simulink model "Solar_Position"  (R2024b)
settings: Solver=FixedStepAuto  StartTime=0.0  StopTime=1200  FixedStep=0.1  RelTol=1e-3
values from neighbouring files (symbols this model uses):
  DayNum = 0    [Inititialisation.m]
  EGlobal = t(2:25, 2:end)    [Inititialisation.m]
  Latitude = 0    [Inititialisation.m]
  Longitude = 0    [Inititialisation.m]
  T_avg = transpose(t(30,2:end))    [Inititialisation.m]
  TimeDiff = 0    [Inititialisation.m]
libraries: simulink_extras x14
settings Model: Creator=Harrison  LastModifiedBy=Harrison
settings DebuggingCC: AlgebraicLoopMsg=none

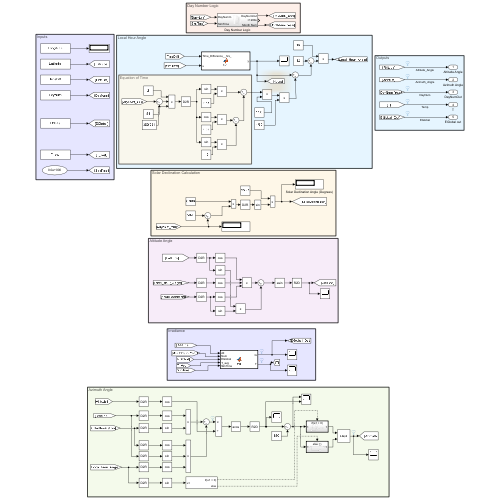
[thumbnail: Simulink's stored preview of the top-level diagram]
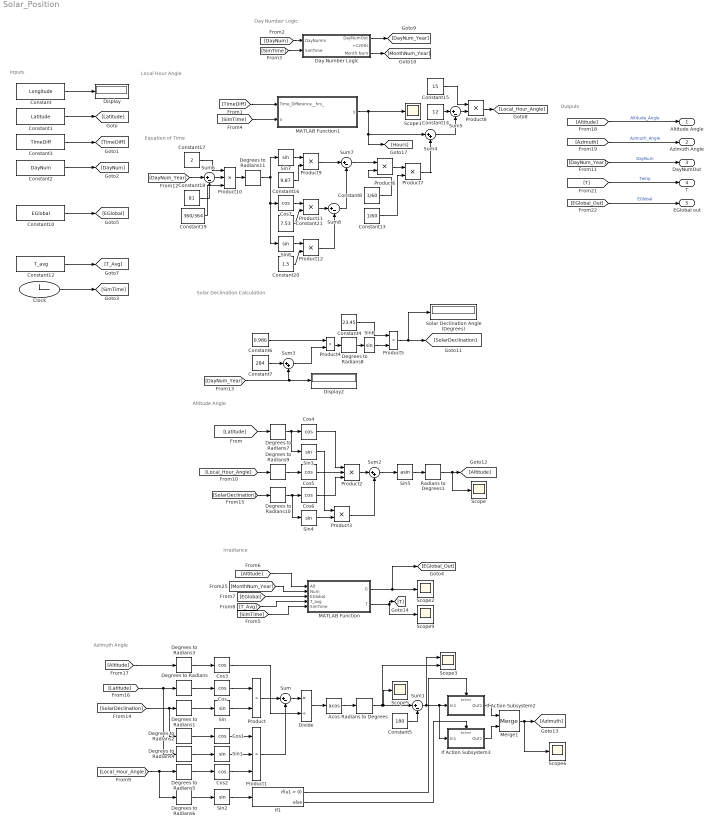
== system Solar_Position ==
  note: Irradiance
  note: Equation of Time
  note: Local Hour Angle
  note: Solar Declination Calculation
  note: Day Number Logic
  note: Altitude Angle
  note: Azimuth Angle
  note: Outputs
  note: Inputs
  Acos : Trigonometry  Operator=acos
  Clock : Clock
      settings: Decimation=100
  Constant : Constant  Value=Longitude
  Constant1 : Constant  Value=Latitude
  Constant10 : Constant  Value=EGlobal
  Constant12 : Constant  Value=T_avg
  Constant13 : Constant  Value=1/60
  Constant14 : Constant  Value=12
  Constant15 : Constant  Value=15
  Constant16 : Constant  Value=9.87
  Constant17 : Constant  Value=2
  Constant18 : Constant  Value=81
  Constant19 : Constant  Value=360/364
  Constant2 : Constant  Value=DayNum
  Constant20 : Constant  Value=1.5
  Constant21 : Constant  Value=7.53
  Constant3 : Constant  Value=TimeDiff
  Constant4 : Constant  Value=23.45
  Constant5 : Constant  Value=180
  Constant6 : Constant  Value=0.986
  Constant7 : Constant  Value=284
  Constant8 : Constant  Value=1/60
  Cos{,1..7} (8 alike) : Trigonometry  Operator=cos
  Day Number Logic : Subsystem
  Degrees to Radians{,1..11} (12 alike) : simulink_extras/Transformations/Degrees to Radians
  Display : Display
  Display2 : Display
  Divide : Product  Inputs=*/
  If Action Subsystem2 : Subsystem  TreatAsAtomicUnit=on
  If Action Subsystem3 : Subsystem  TreatAsAtomicUnit=on
  If1 : If
  MATLAB Function : MATLAB Function  TreatAsAtomicUnit=on
  MATLAB Function1 : MATLAB Function  TreatAsAtomicUnit=on
  Merge1 : Merge
  Product{,3..9,11..12} (10 alike) : Product
  Product1 : Product  Inputs=3
  Product10 : Product  Inputs=3
  Product2 : Product  Inputs=3
  Radians to Degrees : simulink_extras/Transformations/Radians to Degrees
  Radians to Degrees1 : simulink_extras/Transformations/Radians to Degrees
  Scope{,1..2,5..6,9} (6 alike) : Scope
  Scope3 : Scope  NumInputPorts=2
  Sin{,1..4,6..8} (8 alike) : Trigonometry
  Sin5 : Trigonometry  Operator=asin
  Solar Declination Angle (Degrees) : Display
  Sum{,1,5..8} (6 alike) : Sum  Inputs=|+-
  Sum2 : Sum  Inputs=|++
  Sum3 : Sum  Inputs=|++
  Sum4 : Sum  Inputs=|++
  Altitude Angle : Outport
  Azimuth Angle : Outport  Port=2
  DayNumOut : Outport  Port=3
  T : Outport  Port=4
  EGlobal out : Outport  Port=5
  wires:
  Constant/1 -> Display/1
  Radians to Degrees1/1 -> Scope/1, [Altitude]
  Merge1/1 -> Scope6/1, [Azimuth]
  Day Number Logic/1(DayNumOut) -> [DayNum_Year]
  Constant2/1 -> [DayNum]
  MATLAB Function/1(G) -> [EGlobal_Out], Scope2/1
  Constant1/1 -> [Latitude]
  Constant3/1 -> [TimeDiff]
  [DayNum] -> Day Number Logic/1(DayNumIn)
  Clock/1 -> [SimTime]
  [SimTime] -> Day Number Logic/2(SimTime)
  Constant10/1 -> [EGlobal]
  Constant12/1 -> [T_Avg]
  Day Number Logic/3(Month Num) -> [MonthNum_Year]
  [DayNum_Year] -> DayNumOut/1  "DayNum"
  Product8/1 -> [Local_Hour_Angle]
  [Altitude] -> Altitude Angle/1  "Altitude_Angle"
  [Azimuth] -> Azimuth Angle/1  "Azimuth_Angle"
  MATLAB Function/2(T) -> Scope9/1, [T]
  [T] -> T/1  "Temp"
  [EGlobal_Out] -> EGlobal out/1  "EGlobal"
  Degrees to Radians6/1 -> Sin2/1
  Degrees to Radians5/1 -> Cos2/1
  Degrees to Radians4/1 -> Sin1/1
  Degrees to Radians2/1 -> Cos1/1
  Degrees to Radians1/1 -> Sin/1
  Degrees to Radians/1 -> Cos/1
  Constant5/1 -> Sum1/2
  Product/1 -> Sum/1
  Sin/1 -> Product/2
  Cos/1 -> Product/1
  Acos/1 -> Radians to Degrees/1
  Sin1/1 -> Product1/2
  Divide/1 -> Acos/1
  Degrees to Radians3/1 -> Cos3/1
  Sin2/1 -> If1/1
  Cos3/1 -> Divide/2
  Sum/1 -> Divide/1
  If Action Subsystem3/1(Out1) -> Merge1/2
  Cos1/1 -> Product1/1
  Cos2/1 -> Product1/3
  Product1/1 -> Sum/2
  Sum1/1 -> Scope3/1, If Action Subsystem3/1(In1), If Action Subsystem2/1(In1)
  Radians to Degrees/1 -> Sum1/1, Scope5/1, Scope3/2
  If Action Subsystem2/1(Out1) -> Merge1/1
  If1/1 -> If Action Subsystem2/Action
  If1/2 -> If Action Subsystem3/Action
  Degrees to Radians10/1 -> Cos6/1, Sin4/1
  Degrees to Radians9/1 -> Cos5/1
  Degrees to Radians7/1 -> Sin3/1, Cos4/1
  [Local_Hour_Angle] -> Degrees to Radians9/1
  Sum2/1 -> Sin5/1
  Product2/1 -> Sum2/1
  Sin5/1 -> Radians to Degrees1/1
  Product3/1 -> Sum2/2
  Cos6/1 -> Product2/3
  Sin4/1 -> Product3/2
  [Latitude] -> Degrees to Radians7/1
  Sin3/1 -> Product3/1
  Cos5/1 -> Product2/2
  [SolarDeclination] -> Degrees to Radians10/1
  Cos4/1 -> Product2/1
  Sin6/1 -> Product5/2
  Product4/1 -> Degrees to Radians8/1
  Degrees to Radians8/1 -> Sin6/1
  Sum3/1 -> Product4/2
  Constant4/1 -> Product5/1
  Constant6/1 -> Product4/1
  [DayNum_Year] -> Display2/1, Sum3/2
  Constant7/1 -> Sum3/1
  Product5/1 -> Solar Declination Angle (Degrees)/1, [SolarDeclination]
  Sum4/1 -> Sum5/2
  Constant13/1 -> Product7/2
  Product6/1 -> Product7/1
  Sum7/1 -> Product6/1
  Sum5/1 -> Product8/2
  MATLAB Function1/1(y) -> Scope1/1, [Hours], Sum4/1
  Constant14/1 -> Sum5/1
  Product7/1 -> Sum4/2
  Constant8/1 -> Product6/2
  [SimTime] -> MATLAB Function1/2(u)
  Constant15/1 -> Product8/1
  [TimeDiff] -> MATLAB Function1/1(Time_Difference__hrs_)
  [DayNum_Year] -> Sum6/1
  Constant17/1 -> Product10/1
  Product9/1 -> Sum7/1
  Product12/1 -> Sum8/2
  Constant18/1 -> Sum6/2
  Sum6/1 -> Product10/2
  Sin7/1 -> Product9/1
  Product10/1 -> Degrees to Radians11/1
  Sum8/1 -> Sum7/2
  Constant16/1 -> Product9/2
  Cos7/1 -> Product11/1
  Constant21/1 -> Product11/2
  Product11/1 -> Sum8/1
  Degrees to Radians11/1 -> Sin8/1, Cos7/1, Sin7/1
  Constant20/1 -> Product12/2
  Sin8/1 -> Product12/1
  Constant19/1 -> Product10/3
  [SimTime] -> MATLAB Function/5(SimTime)
  [T_Avg] -> MATLAB Function/4(T_avg)
  [EGlobal] -> MATLAB Function/3(EGlobal)
  [MonthNum_Year] -> MATLAB Function/2(Num)
  [Altitude] -> MATLAB Function/1(Alt)
  [SolarDeclination] -> Degrees to Radians2/1, Degrees to Radians1/1
  [Local_Hour_Angle] -> Degrees to Radians6/1, Degrees to Radians5/1
  [Altitude] -> Degrees to Radians3/1
  [Latitude] -> Degrees to Radians4/1, Degrees to Radians/1

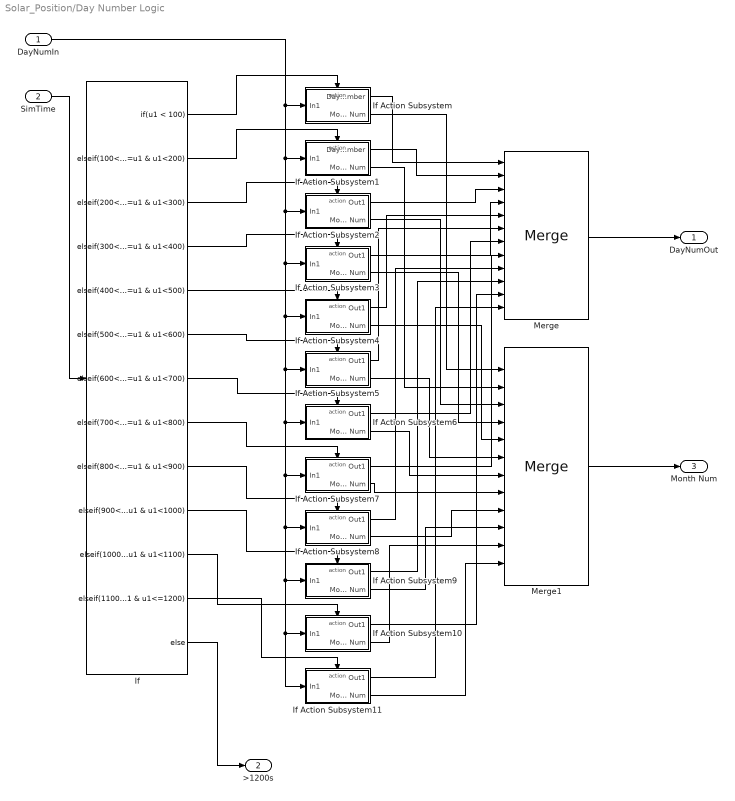
== system Solar_Position/Day Number Logic ==
  DayNumIn : Inport
  SimTime : Inport  Port=2
  If : If  IfExpression=u1 < 100  ElseIfExpressions=100<=u1 & u1<200, 200<=u1 & u1<300, 300<=u1 & u1<400, 400<=u1 & u1<500, 500<=u1 & u1<600, 600<=u1 & u1<700, 700<=u1 & u1<800, 800<=u1 & u1<900, 900<=u1 & u1<1000, 1000<=u1 & u1<1100, 1100<=u1 & u1<=1200
  If Action Subsystem : Subsystem  TreatAsAtomicUnit=on
  If Action Subsystem1 : Subsystem  TreatAsAtomicUnit=on
  If Action Subsystem10 : Subsystem  TreatAsAtomicUnit=on
  If Action Subsystem11 : Subsystem  TreatAsAtomicUnit=on
  If Action Subsystem2 : Subsystem  TreatAsAtomicUnit=on
  If Action Subsystem3 : Subsystem  TreatAsAtomicUnit=on
  If Action Subsystem4 : Subsystem  TreatAsAtomicUnit=on
  If Action Subsystem5 : Subsystem  TreatAsAtomicUnit=on
  If Action Subsystem6 : Subsystem  TreatAsAtomicUnit=on
  If Action Subsystem7 : Subsystem  TreatAsAtomicUnit=on
  If Action Subsystem8 : Subsystem  TreatAsAtomicUnit=on
  If Action Subsystem9 : Subsystem  TreatAsAtomicUnit=on
  Merge : Merge  Inputs=12
  Merge1 : Merge  Inputs=12
  DayNumOut : Outport
  >1200s : Outport  Port=2
  Month Num : Outport  Port=3
  wires:
  If/8 -> If Action Subsystem7/Action
  If/5 -> If Action Subsystem4/Action
  DayNumIn/1 -> If Action Subsystem11/1(In1), If Action Subsystem10/1(In1), If Action Subsystem9/1(In1), If Action Subsystem8/1(In1), If Action Subsystem7/1(In1), If Action Subsystem6/1(In1), If Action Subsystem5/1(In1), If Action Subsystem4/1(In1), If Action Subsystem3/1(In1), If Action Subsystem2/1(In1), If Action Subsystem1/1(In1), If Action Subsystem/1(In1)
  If Action Subsystem/1(Day number) -> Merge/1
  If Action Subsystem10/1(Out1) -> Merge/11
  If Action Subsystem5/1(Out1) -> Merge/6
  If Action Subsystem11/1(Out1) -> Merge/12
  If Action Subsystem8/1(Out1) -> Merge/9
  If/10 -> If Action Subsystem9/Action
  If Action Subsystem6/1(Out1) -> Merge/7
  If/7 -> If Action Subsystem6/Action
  If/11 -> If Action Subsystem10/Action
  If/1 -> If Action Subsystem/Action
  If Action Subsystem7/1(Out1) -> Merge/8
  If/3 -> If Action Subsystem2/Action
  If/12 -> If Action Subsystem11/Action
  If Action Subsystem2/1(Out1) -> Merge/3
  If/6 -> If Action Subsystem5/Action
  If Action Subsystem4/1(Out1) -> Merge/5
  If/2 -> If Action Subsystem1/Action
  If Action Subsystem9/1(Out1) -> Merge/10
  If Action Subsystem3/1(Out1) -> Merge/4
  If/9 -> If Action Subsystem8/Action
  If Action Subsystem1/1(Day number) -> Merge/2
  If/4 -> If Action Subsystem3/Action
  Merge/1 -> DayNumOut/1
  SimTime/1 -> If/1
  If/13 -> >1200s/1
  If Action Subsystem/2(Month Num) -> Merge1/1
  If Action Subsystem1/2(Month Num) -> Merge1/2
  If Action Subsystem2/2(Month Num) -> Merge1/3
  If Action Subsystem3/2(Month Num) -> Merge1/4
  If Action Subsystem4/2(Month Num) -> Merge1/5
  If Action Subsystem5/2(Month Num) -> Merge1/6
  If Action Subsystem6/2(Month Num) -> Merge1/7
  If Action Subsystem7/2(Month Num) -> Merge1/8
  If Action Subsystem8/2(Month Num) -> Merge1/9
  If Action Subsystem9/2(Month Num) -> Merge1/10
  If Action Subsystem10/2(Month Num) -> Merge1/11
  If Action Subsystem11/2(Month Num) -> Merge1/12
  Merge1/1 -> Month Num/1

== system Solar_Position/If Action Subsystem2 ==
  In1 : Inport
  Action Port : ActionPort  ActionPortLabel=if(u1 > 0)
  Constant : Constant  Value=-1
  Product : Product
  Scope : Scope
  Out1 : Outport
  wires:
  In1/1 -> Scope/1, Product/1
  Product/1 -> Out1/1
  Constant/1 -> Product/2

== system Solar_Position/If Action Subsystem3 ==
  In1 : Inport
  Action Port : ActionPort  ActionPortLabel=else
  Scope : Scope
  Out1 : Outport
  wires:
  In1/1 -> Scope/1, Out1/1

== system Solar_Position/Day Number Logic/If Action Subsystem ==
  In1 : Inport
  Action Port : ActionPort  ActionPortLabel=if(u1 < 100)
  Constant : Constant
  Day number : Outport
  Month Num : Outport  Port=2
  wires:
  In1/1 -> Day number/1
  Constant/1 -> Month Num/1

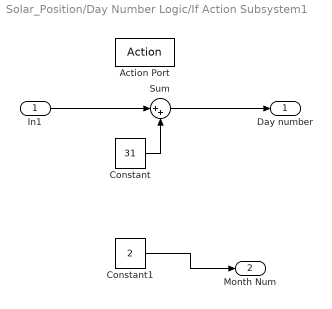
== system Solar_Position/Day Number Logic/If Action Subsystem1 ==
  In1 : Inport
  Action Port : ActionPort  ActionPortLabel=elseif(100<=u1 & u1<200)
  Constant : Constant  Value=31
  Constant1 : Constant  Value=2
  Sum : Sum  Inputs=|++
  Day number : Outport
  Month Num : Outport  Port=2
  wires:
  In1/1 -> Sum/1
  Sum/1 -> Day number/1
  Constant/1 -> Sum/2
  Constant1/1 -> Month Num/1

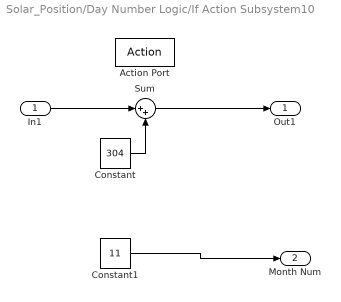
== system Solar_Position/Day Number Logic/If Action Subsystem10 ==
  In1 : Inport
  Action Port : ActionPort  ActionPortLabel=elseif( 1000<=u1 & u1<1100)
  Constant : Constant  Value=304
  Constant1 : Constant  Value=11
  Sum : Sum  Inputs=|++
  Out1 : Outport
  Month Num : Outport  Port=2
  wires:
  In1/1 -> Sum/1
  Sum/1 -> Out1/1
  Constant/1 -> Sum/2
  Constant1/1 -> Month Num/1

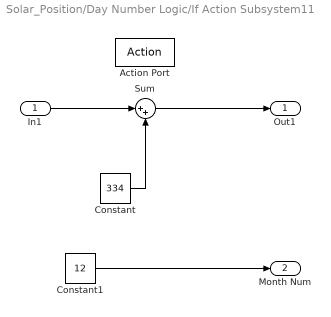
== system Solar_Position/Day Number Logic/If Action Subsystem11 ==
  In1 : Inport
  Action Port : ActionPort  ActionPortLabel=elseif( 1100<=u1 & u1<=1200)
  Constant : Constant  Value=334
  Constant1 : Constant  Value=12
  Sum : Sum  Inputs=|++
  Out1 : Outport
  Month Num : Outport  Port=2
  wires:
  In1/1 -> Sum/1
  Sum/1 -> Out1/1
  Constant/1 -> Sum/2
  Constant1/1 -> Month Num/1

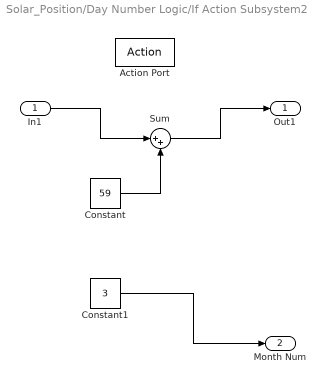
== system Solar_Position/Day Number Logic/If Action Subsystem2 ==
  In1 : Inport
  Action Port : ActionPort  ActionPortLabel=elseif( 200<=u1 & u1<300)
  Constant : Constant  Value=59
  Constant1 : Constant  Value=3
  Sum : Sum  Inputs=|++
  Out1 : Outport
  Month Num : Outport  Port=2
  wires:
  In1/1 -> Sum/1
  Sum/1 -> Out1/1
  Constant/1 -> Sum/2
  Constant1/1 -> Month Num/1

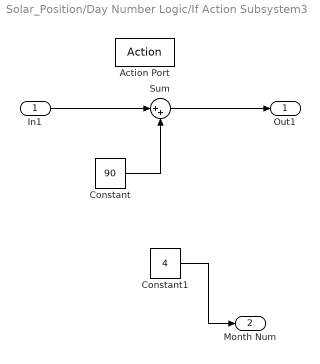
== system Solar_Position/Day Number Logic/If Action Subsystem3 ==
  In1 : Inport
  Action Port : ActionPort  ActionPortLabel=elseif( 300<=u1 & u1<400)
  Constant : Constant  Value=90
  Constant1 : Constant  Value=4
  Sum : Sum  Inputs=|++
  Out1 : Outport
  Month Num : Outport  Port=2
  wires:
  In1/1 -> Sum/1
  Sum/1 -> Out1/1
  Constant/1 -> Sum/2
  Constant1/1 -> Month Num/1

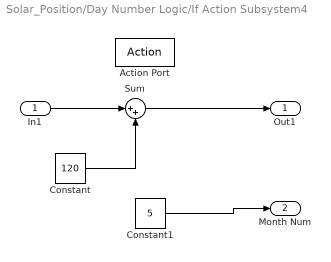
== system Solar_Position/Day Number Logic/If Action Subsystem4 ==
  In1 : Inport
  Action Port : ActionPort  ActionPortLabel=elseif( 400<=u1 & u1<500)
  Constant : Constant  Value=120
  Constant1 : Constant  Value=5
  Sum : Sum  Inputs=|++
  Out1 : Outport
  Month Num : Outport  Port=2
  wires:
  In1/1 -> Sum/1
  Sum/1 -> Out1/1
  Constant/1 -> Sum/2
  Constant1/1 -> Month Num/1

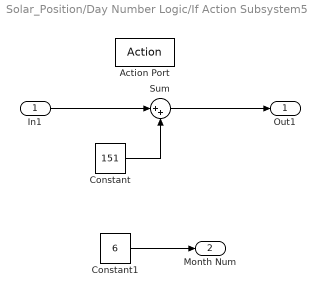
== system Solar_Position/Day Number Logic/If Action Subsystem5 ==
  In1 : Inport
  Action Port : ActionPort  ActionPortLabel=elseif( 500<=u1 & u1<600)
  Constant : Constant  Value=151
  Constant1 : Constant  Value=6
  Sum : Sum  Inputs=|++
  Out1 : Outport
  Month Num : Outport  Port=2
  wires:
  In1/1 -> Sum/1
  Sum/1 -> Out1/1
  Constant/1 -> Sum/2
  Constant1/1 -> Month Num/1

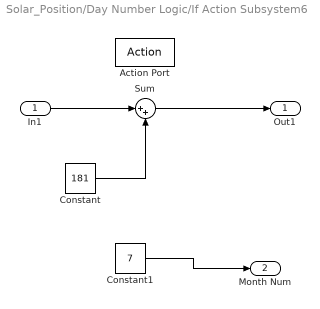
== system Solar_Position/Day Number Logic/If Action Subsystem6 ==
  In1 : Inport
  Action Port : ActionPort  ActionPortLabel=elseif( 600<=u1 & u1<700)
  Constant : Constant  Value=181
  Constant1 : Constant  Value=7
  Sum : Sum  Inputs=|++
  Out1 : Outport
  Month Num : Outport  Port=2
  wires:
  In1/1 -> Sum/1
  Sum/1 -> Out1/1
  Constant/1 -> Sum/2
  Constant1/1 -> Month Num/1

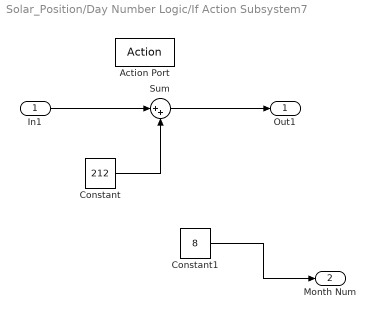
== system Solar_Position/Day Number Logic/If Action Subsystem7 ==
  In1 : Inport
  Action Port : ActionPort  ActionPortLabel=elseif( 700<=u1 & u1<800)
  Constant : Constant  Value=212
  Constant1 : Constant  Value=8
  Sum : Sum  Inputs=|++
  Out1 : Outport
  Month Num : Outport  Port=2
  wires:
  In1/1 -> Sum/1
  Sum/1 -> Out1/1
  Constant/1 -> Sum/2
  Constant1/1 -> Month Num/1

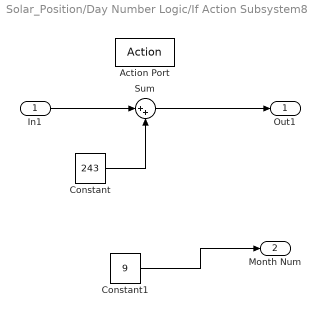
== system Solar_Position/Day Number Logic/If Action Subsystem8 ==
  In1 : Inport
  Action Port : ActionPort  ActionPortLabel=elseif( 800<=u1 & u1<900)
  Constant : Constant  Value=243
  Constant1 : Constant  Value=9
  Sum : Sum  Inputs=|++
  Out1 : Outport
  Month Num : Outport  Port=2
  wires:
  Sum/1 -> Out1/1
  In1/1 -> Sum/1
  Constant/1 -> Sum/2
  Constant1/1 -> Month Num/1

== system Solar_Position/Day Number Logic/If Action Subsystem9 ==
  In1 : Inport
  Action Port : ActionPort  ActionPortLabel=elseif( 900<=u1 & u1<1000)
  Constant : Constant  Value=273
  Constant1 : Constant  Value=10
  Sum : Sum  Inputs=|++
  Out1 : Outport
  Month Num : Outport  Port=2
  wires:
  In1/1 -> Sum/1
  Sum/1 -> Out1/1
  Constant/1 -> Sum/2
  Constant1/1 -> Month Num/1

== matlab function Solar_Position/MATLAB Function ==
  data: Alt input; G output; Num input; EGlobal input; T_avg input; T output; SimTime input
function [G, T] = fcn(Alt, Num, EGlobal, T_avg, SimTime)
T = T_avg(Num);
N = ((SimTime - (100 * (Num - 1))) * 24) / 100;
N = floor(N+1);
if Alt <= 0
    G = 0
else
    if N == 25
        G = 0;
    else
        G = EGlobal(N ,Num);
    
    end
end

== matlab function Solar_Position/MATLAB Function1 ==
  data: Time_Difference__hrs_ input; u input; y output
function y = fcn(Time_Difference__hrs_, u)
diff = Time_Difference__hrs_/100;
a = u/100;
b = a + diff;
y = mod((24 * b),24);
